simulink model "simulink_model"  (R2025b)
settings: Solver=VariableStepAuto  StartTime=0.0  StopTime=10.0  RelTol=1e-3
values from neighbouring files (symbols this model uses):
  G = 6.6743 * 10 ^ -11    (= 6.6743e-11)    [matlab_model.m]
  mass1 = 5.972 * 10 ^ 24    (= 5.972e+24)    [matlab_model.m]
  mass2 = 7.348 * 10 ^ 6    (= 7348000)    [matlab_model.m]
settings Model: Creator=leonard  LastModifiedBy=leonard

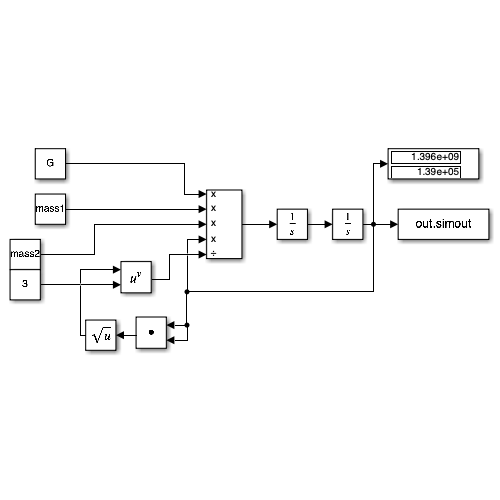
[thumbnail: Simulink's stored preview of the top-level diagram]
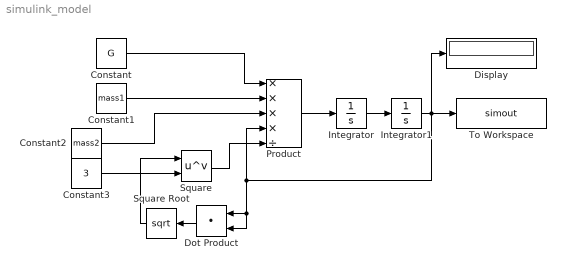
== system simulink_model ==
  Constant : Constant  Value=G
  Constant1 : Constant  Value=mass1
  Constant2 : Constant  Value=mass2
  Constant3 : Constant  Value=3
  Display : Display
  Dot Product : DotProduct  OutDataTypeStr=Inherit: Inherit via internal rule
  Integrator : Integrator  InitialCondition=[0,6960]
  Integrator1 : Integrator  InitialCondition=[300000,0]
  Product : Product  Inputs=****/
  Square : Math  Operator=pow
  Square Root : Sqrt
  To Workspace : ToWorkspace  VariableName=simout  SaveFormat=Timeseries  SampleTime=-1
  wires:
  Integrator/1 -> Integrator1/1
  Constant/1 -> Product/1
  Constant1/1 -> Product/2
  Constant2/1 -> Product/3
  Integrator1/1 -> To Workspace/1, Display/1, Dot Product/2, Dot Product/1, Product/4
  Square/1 -> Product/5
  Product/1 -> Integrator/1
  Square Root/1 -> Square/1
  Constant3/1 -> Square/2
  Dot Product/1 -> Square Root/1
